simulink model "FeedForward"  (R2018b)
settings: Solver=ode1  StartTime=0.0  StopTime=1000  FixedStep=1  RelTol=1e-3
libraries: FMIKit_blocks x1
settings Model: Creator=U370698  LastModifiedBy=U375749
settings DebuggingCC: LibraryContextMissingDiagnostic=none
settings SFSimCC: SimUseLocalCustomCode=off
settings RTWCC: RTWUseLocalCustomCode=off

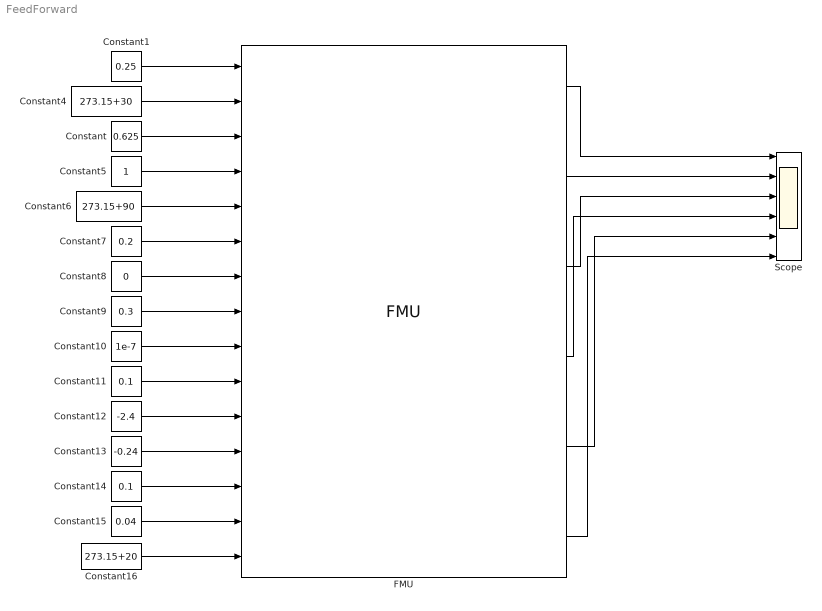
== system FeedForward ==
  Constant : Constant  Value=0.625
  Constant1 : Constant  Value=0.25
  Constant10 : Constant  Value=1e-7
  Constant11 : Constant  Value=0.1
  Constant12 : Constant  Value=-2.4
  Constant13 : Constant  Value=-0.24
  Constant14 : Constant  Value=0.1
  Constant15 : Constant  Value=0.04
  Constant16 : Constant  Value=273.15+20
  Constant4 : Constant  Value=273.15+30
  Constant5 : Constant
  Constant6 : Constant  Value=273.15+90
  Constant7 : Constant  Value=0.2
  Constant8 : Constant  Value=0
  Constant9 : Constant  Value=0.3
  FMU : FMIKit_blocks/FMU  SFunctionModules=''
      settings: SourceProductName=FMI Kit
  Scope : Scope  NumInputPorts=6
  wires:
  Constant1/1 -> FMU/1
  Constant4/1 -> FMU/2
  Constant/1 -> FMU/3
  Constant5/1 -> FMU/4
  Constant6/1 -> FMU/5
  Constant8/1 -> FMU/7
  Constant9/1 -> FMU/8
  Constant10/1 -> FMU/9
  Constant11/1 -> FMU/10
  Constant12/1 -> FMU/11
  Constant13/1 -> FMU/12
  Constant14/1 -> FMU/13
  Constant15/1 -> FMU/14
  Constant16/1 -> FMU/15
  Constant7/1 -> FMU/6
  FMU/2 -> Scope/2
  FMU/3 -> Scope/3
  FMU/1 -> Scope/1
  FMU/4 -> Scope/4
  FMU/5 -> Scope/5
  FMU/6 -> Scope/6
